simulink model "Mazesolving_nic2"  (R2023a)
settings: Solver=FixedStepDiscrete  StartTime=0.0  StopTime=inf  FixedStep=0.01  RelTol=1e-3  EnableMultiTasking=on
undefined symbols (not defined in the file or in its folder): InputPWM, WheelSpeed
libraries: arduinolib x10, simulink x2, mobileRoboticsTrainingLib x1, arduinosensorlib x1
settings Model: ExtModeTrigDuration=2  Creator=thuto  LastModifiedBy=thuto
settings OptimizationCC: EnhancedBackFolding=on  PassReuseOutputArgsAs=Individual arguments  ZeroExternalMemoryAtStartup=off  ZeroInternalMemoryAtStartup=off  MaxStackSize=64  OptimizeBlockOrder=speed  DifferentSizesBufferReuse=on  OptimizationCustomize=off  EfficientTunableParamExpr=on
settings DebuggingCC: ParameterTunabilityLossMsg=error
settings HardwareCC: ProdBitPerPointer=32  ProdBitPerSizeT=32  ProdBitPerPtrDiffT=32  ProdLargestAtomicInteger=Long  ProdLargestAtomicFloat=Double  ProdWordSize=32  ProdHWDeviceType=ARM Compatible->ARM Cortex  UseEmbeddedCoderFeatures=off
settings SFSimCC: MATLABDynamicMemAlloc=off
settings RTWCC: Description=Embedded Coder  SystemTargetFile=ert.tlc  HardwareBoard=Arduino Nano 33 IoT  TemplateMakefile=ert_default_tmf  Toolchain=Arduino ARM  BuildConfiguration=Faster Runs
settings CodeAppCC: ForceParamTrailComments=on  IgnoreCustomStorageClasses=off  OperatorAnnotations=on  SimulinkDataObjDesc=on  SFDataObjDesc=on  InsertBlockDesc=on
settings ERTTargetCC: SupportContinuousTime=on  SupportNonInlinedSFcns=on  SupportVariableSizeSignals=on  ExtModeTransport=3  ExtModeStaticAlloc=on  ExtModeAutomaticAllocSize=off  ExtModeStaticAllocSize=8192  ExtModeMexFile=ext_xcp  ExtModeIntrfLevel=Level2 - Open

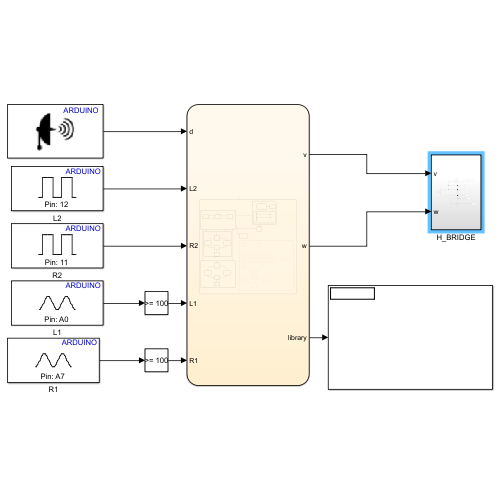
[thumbnail: Simulink's stored preview of the top-level diagram]
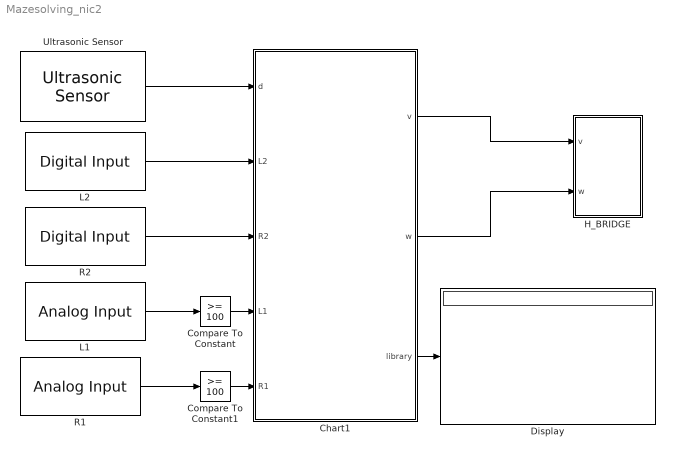
== system Mazesolving_nic2 ==
  Chart1 : Stateflow chart  TreatAsAtomicUnit=on
      settings: PortSchema="{\"entries\":[{\"content\":{\"sides\":[{\"content\":{\"connectorIds\":[\"In1\",\"In2\",\"In3\",\"In4\",\"In5\"]},\"type\":\"ConnectorPlacement.EquallySpacedRectSide\",\"uuid\":\"8989f916-8415-435d-af3d-fcc60b5fc6ff\"},{\"content\":{\"connectorIds\":[\"Out2\",\"Out1\",\"Out3\"],\"side\":\"RIGHT\"},\"type\":\"ConnectorPlacement.EquallySpacedRectSide\",\"uuid\":\"e98c1212-df50-4216-8d0f-99e5b5b5ad95\"},{\"content\":{\"side\":\"TOP\"},\"type\":\"ConnectorPlacement.EquallySpacedRectSide\",\"uuid\":\"10937b35-4214-45c4-b9a2-486c2e88bca2\"}]},\"type\":\"ConnectorPlacement.EquallySpacedConnector\",\"uuid\":\"7f4a8ad6-df0f-4819-a42c-ce6b812eb228\"}],\"packageUris\":[\"http://schema.mathworks.com/mf0/Connector/R2020b\"],\"version\":\"1.0\"}"
  Compare To Constant : simulink/Logic and Bit Operations/Compare To Constant  relop=>=  const=100  OutDataTypeStr=boolean
  Compare To Constant1 : simulink/Logic and Bit Operations/Compare To Constant  relop=>=  const=100  OutDataTypeStr=boolean
  Display : Display
  H_BRIDGE : Subsystem
  L1 : arduinolib/Analog Input  pinNumber=0  ReadResultsOnly=off  ConversionTriggerSource=Software  ExternalTriggerType=uint32( 0 )  OutputDataType=uint16  EnableConversionCompleteNotify=off  EnableOuputStatus=off  SampleTime=0.01  blockPlatform=arduino
  L2 : arduinolib/Digital Input  pinNumber=12  mode=Default  Direction=input  SampleTime=0.01  blockPlatform=arduino
  R1 : arduinolib/Analog Input  pinNumber=7  ReadResultsOnly=off  ConversionTriggerSource=Software  ExternalTriggerType=uint32( 0 )  OutputDataType=uint16  EnableConversionCompleteNotify=off  EnableOuputStatus=off  SampleTime=0.01  blockPlatform=arduino
  R2 : arduinolib/Digital Input  pinNumber=11  mode=Default  Direction=input  SampleTime=0.01  blockPlatform=arduino
  Ultrasonic Sensor : arduinosensorlib/Ultrasonic Sensor  NumSignalPins=2  TrigPin=9  EchoPin=10  SignalPin=3  SampleTime_=0.01  blockPlatform=ARDUINO
  wires:
  Chart1/3(library) -> Display/1
  Chart1/2(v) -> H_BRIDGE/1(v)
  Chart1/1(w) -> H_BRIDGE/2(w)
  L2/1 -> Chart1/2(L2)
  R2/1 -> Chart1/3(R2)
  L1/1 -> Compare To Constant/1
  Compare To Constant/1 -> Chart1/4(L1)
  R1/1 -> Compare To Constant1/1
  Compare To Constant1/1 -> Chart1/5(R1)
  Ultrasonic Sensor/1 -> Chart1/1(d)

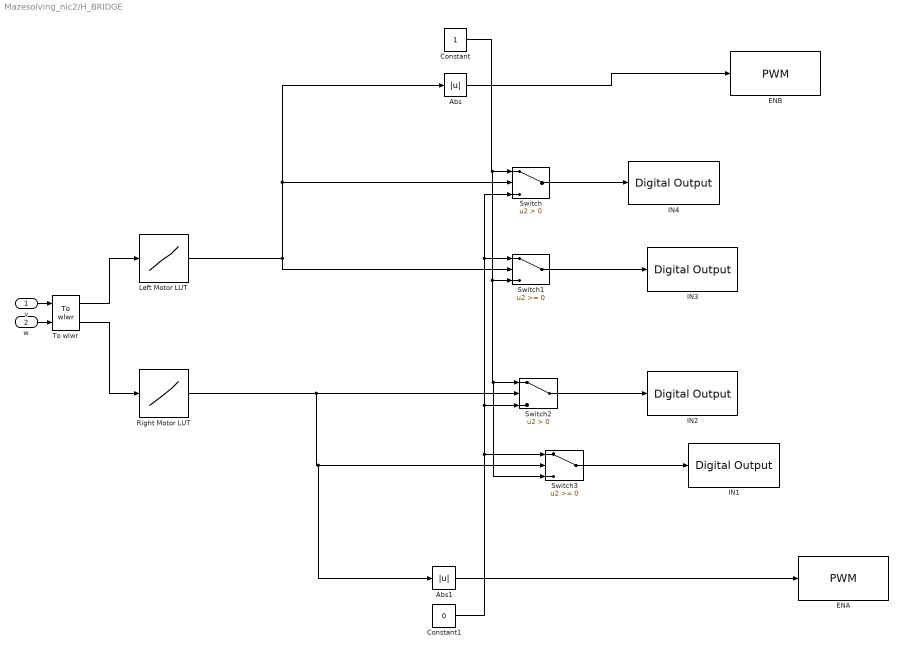
== system Mazesolving_nic2/H_BRIDGE ==
  v : Inport
  w : Inport  Port=2
  Abs : Abs  SaturateOnIntegerOverflow=off
  Abs1 : Abs  SaturateOnIntegerOverflow=off
  Constant : Constant
  Constant1 : Constant  Value=0
  ENA : arduinolib/PWM  pinNumber=16  frequencyType=Default  desiredFrequency=490.2  achievableFrequency=490.2
  ENB : arduinolib/PWM  pinNumber=17  frequencyType=Default  desiredFrequency=490.2  achievableFrequency=490.2
  IN1 : arduinolib/Digital Output  pinNumber=5  Direction=output  blockPlatform=arduino
  IN2 : arduinolib/Digital Output  pinNumber=8  Direction=output  blockPlatform=arduino
  IN3 : arduinolib/Digital Output  pinNumber=7  Direction=output  blockPlatform=arduino
  IN4 : arduinolib/Digital Output  pinNumber=6  Direction=output  blockPlatform=arduino
  Left Motor LUT : Lookup_n-D  NumberOfTableDimensions=1  BreakpointsForDimension1=WheelSpeed  Table=InputPWM  InterpMethod=Nearest  ExtrapMethod=Clip  InternalRulePriority=Speed  RndMeth=Simplest
  Right Motor LUT : Lookup_n-D  NumberOfTableDimensions=1  BreakpointsForDimension1=WheelSpeed  Table=InputPWM  InterpMethod=Nearest  ExtrapMethod=Clip  InternalRulePriority=Speed  RndMeth=Simplest
  Switch : Switch  Criteria=u2 > Threshold  SaturateOnIntegerOverflow=off  InputSameDT=off
  Switch1 : Switch  SaturateOnIntegerOverflow=off  InputSameDT=off
  Switch2 : Switch  Criteria=u2 > Threshold  SaturateOnIntegerOverflow=off  InputSameDT=off
  Switch3 : Switch  SaturateOnIntegerOverflow=off  InputSameDT=off
  To wlwr : mobileRoboticsTrainingLib/To wlwr  axleLength=axleLength  wheelR=wheelR
  wires:
  Switch3/1 -> IN1/1
  Switch2/1 -> IN2/1
  Switch/1 -> IN4/1
  Switch1/1 -> IN3/1
  Constant/1 -> Switch/1, Switch1/3, Switch2/1, Switch3/3
  Left Motor LUT/1 -> Switch1/2, Switch/2, Abs/1
  Right Motor LUT/1 -> Switch2/2, Abs1/1, Switch3/2
  Constant1/1 -> Switch/3, Switch1/1, Switch2/3, Switch3/1
  To wlwr/1 -> Left Motor LUT/1
  v/1 -> To wlwr/1
  To wlwr/2 -> Right Motor LUT/1
  w/1 -> To wlwr/2
  Abs1/1 -> ENA/1
  Abs/1 -> ENB/1

== stateflow chart Mazesolving_nic2/Chart1 ==
  state mazeSolving
    entry:
    n=1;
    library = zeros(5);
    vDefault=0.2;
    detect=0;
    closest=1;
    state detect
      entry:
      v=0;
      w=0;
      exit:
      n=n+1;
      state measure
        entry:
        library(n)=d;
      state exit
        entry:
        detect = 1;
      state closest
        (default) -> (junction 212)
        (junction 212) -> (junction 214) [order 1] : [d>0 && d<library(n-1) ]
        (junction 212) -> (junction 218) [order 2] : {closest=closest}
        (junction 214) -> (junction 216) : {closest=n}
        (junction 216) -> (junction 218)
        (junction 218) -> (junction 226)
      (default) -> measure
      measure -> exit [order 2] : after(1, sec)
      closest -> exit : after(1, sec)
      measure -> closest [order 1] : [n>1]
    state lineFollowing
      state goCW
        entry:
        w = -10;
        v=vDefault;
      state goStraight
        entry:
        w = 0;
        v=vDefault;
      state goCCW
        entry:
        w = 10;
        v=vDefault;
      (default) -> mazeSolving.lineFollowing.goStraight
      mazeSolving.lineFollowing.goCW -> mazeSolving.lineFollowing.goStraight : [L1==0]
      mazeSolving.lineFollowing.goCCW -> mazeSolving.lineFollowing.goStraight : [R1==0]
      mazeSolving.lineFollowing.goStraight -> mazeSolving.lineFollowing.goCW [order 2] : [L1==1]
      mazeSolving.lineFollowing.goStraight -> mazeSolving.lineFollowing.goCCW [order 1] : [R1==1]
    state turn180
      entry:
      during:
      v=0;
      w=-1;
    state turn
      state startTurn
        entry:
        turn=0;
        w=0;
        v=0.01;
      state CW
        during:
        w=1;
        exit:
        branchDirec=1;
      state CCW
        during:
        w=-1;
        exit:
        branchDirec=-1;
      state turn
        exit:
        turn=1;
      state endTurn
      (default) -> mazeSolving.turn.startTurn
      mazeSolving.turn.startTurn -> mazeSolving.turn.CCW [order 1] : [R2==0]
      mazeSolving.turn.startTurn -> mazeSolving.turn.CW [order 2] : [L2==0]
      mazeSolving.turn.CW -> mazeSolving.turn.turn : [L1==1 && R1==1]
      mazeSolving.turn.CCW -> mazeSolving.turn.turn : [L1==1 && R1==1]
      mazeSolving.turn.turn -> mazeSolving.turn.endTurn : [L1==0 && R1 ==0]
    state end
      entry:
      v=0;
      w=0;
    state return [commented out]
      entry:
      state startTurn [commented out]
        during:
        v=0;
        w=-50;
      state endTurn [commented out]
        during:
        v=0;
        w=-50;
      state returnLineFollowing [commented out]
        state goCW [commented out]
          entry:
          w = -50;
          v=vDefault;
        state goStraight [commented out]
          entry:
          w = 0;
          v=vDefault;
        state goCCW [commented out]
          entry:
          w = 50;
          v=vDefault;
        (default) -> mazeSolving.return.returnLineFollowing.goStraight [commented out]
        mazeSolving.return.returnLineFollowing.goCW -> mazeSolving.return.returnLineFollowing.goStraight [commented out] : [L1==0]
        mazeSolving.return.returnLineFollowing.goCCW -> mazeSolving.return.returnLineFollowing.goStraight [commented out] : [R1==0]
        mazeSolving.return.returnLineFollowing.goStraight -> mazeSolving.return.returnLineFollowing.goCW [commented out] : [L1==1]
        mazeSolving.return.returnLineFollowing.goStraight -> mazeSolving.return.returnLineFollowing.goCCW [commented out] : [R1==1]
      state stop [commented out]
        entry:
        v=0;
        w=0;
      state wait [commented out]
        entry:
        v=vDefault;
      state countBranches [commented out]
        exit:
        n=n-1;
      state turnRight [commented out]
        during:
        v=vDefault;
        w=-50;
        exit:
        branchDirec=-1;
      state startBranch [commented out]
        entry:
        detect=0;
      state endJoinBranch [commented out]
        entry:
        turn=1;
      state turnLeft [commented out]
        during:
        v=vDefault;
        w=50;
        exit:
        branchDirec=1;
      (default) -> mazeSolving.return.startTurn [commented out]
      mazeSolving.return.startTurn -> mazeSolving.return.endTurn [commented out] : [L1==1 && R1==1]
      mazeSolving.return.endTurn -> returnLineFollowing [commented out] : [L1==0 && R1==0]
      returnLineFollowing -> stop [commented out] : [R1==1 && L1==1]
      returnLineFollowing -> wait [commented out] : [xor(R2==0, L2==0)]
      countBranches -> returnLineFollowing [commented out] : [(n-1)>closest]
      endJoinBranch -> returnLineFollowing [commented out] : [turn==1]
      wait -> startBranch [commented out] : [(n-1)==closest]
      wait -> countBranches [commented out] : [R2==1 && L2==1]
      startBranch -> turnRight [commented out] : [R2==0]
      turnRight -> endJoinBranch [commented out] : [theta<=3]
      startBranch -> turnLeft [commented out] : [L2==0]
      turnLeft -> endJoinBranch [commented out] : [theta<=0.1 && theta>=0]
    state joinMain
      state startMain
        entry:
        turn=0;
        v=0;
        w=0;
      state CW
        during:
        w=5;
        exit:
        branchDirec=0;
      state CCW
        during:
        w=-5;
        exit:
        branchDirec=0;
      state turn
        exit:
        turn=1;
        detect=0;
      state endTurn
      (default) -> startMain
      startMain -> mazeSolving.joinMain.CCW [order 1] : [branchDirec==-1]
      startMain -> mazeSolving.joinMain.CW [order 2] : [branchDirec==1]
      mazeSolving.joinMain.CW -> mazeSolving.joinMain.turn : [L1==1 && R1==1]
      mazeSolving.joinMain.CCW -> mazeSolving.joinMain.turn : [L1==1 && R1==1]
      mazeSolving.joinMain.turn -> mazeSolving.joinMain.endTurn : [L1==0 && R1 ==0]
    (default) -> lineFollowing
    lineFollowing -> detect [order 1] : [R1==1 && L1==1]
    detect -> turn180 : [detect==1]
    lineFollowing -> end [order 3] : [R1==0 && L1==0 && R2==0 && L2==0]
    turn180 -> lineFollowing : [R1==0 && L1==0]
    lineFollowing -> joinMain [order 4] : [R1==1 && L1==1 && detect==1]
    lineFollowing -> mazeSolving.turn [order 2] : [xor(R2==0, L2==0)]
    mazeSolving.turn -> lineFollowing : [turn==1]
    joinMain -> lineFollowing : [turn==1]
    end -> return [commented out]
  (default) -> mazeSolving
  data: w output; v output; vDefault local =0.2; n local; turn local; detect local; branchDirec local; library output; d input =1; closest local; L2 input; R2 input; L1 input; R1 input
